simulink model "model1"  (R2023b)
settings: Solver=VariableStepAuto  StartTime=0.0  StopTime=8  RelTol=1e-3
model workspace (MAT data in the model file):
  T = Simulink.Parameter
  T.Value = 1
  T.DataType = 'auto'
  T.Complexity = 'real'
  T.Dimensions = [1 1]
  k = 1
  op = 2
settings Model: Creator=kacpe  LastModifiedBy=kacpe
settings DataIOCC: ReturnWorkspaceOutputs=off

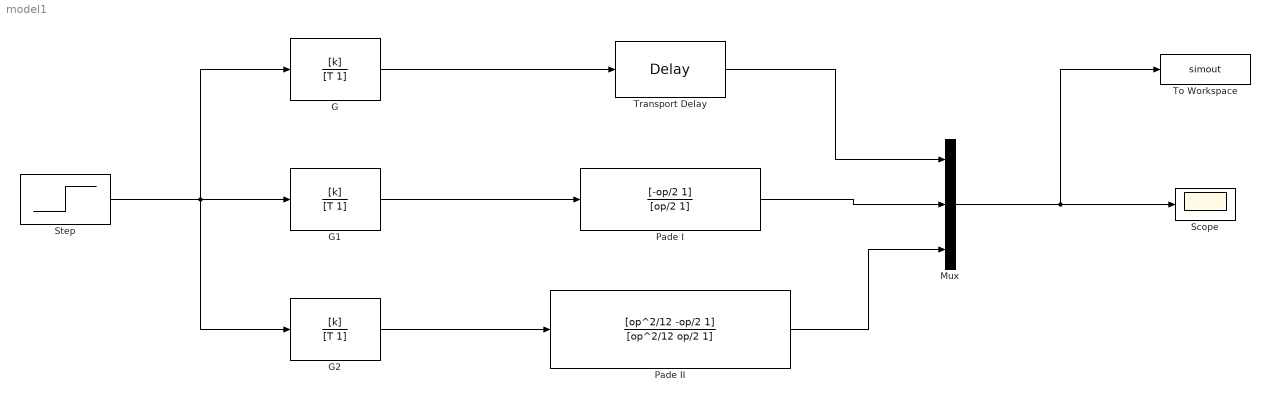
== system model1 ==
  G : TransferFcn  Numerator=[k]  Denominator=[T 1]
  G1 : TransferFcn  Numerator=[k]  Denominator=[T 1]
  G2 : TransferFcn  Numerator=[k]  Denominator=[T 1]
  Mux : Mux  Inputs=3
  Pade I : TransferFcn  Numerator=[-op/2 1]  Denominator=[op/2 1]
  Pade II : TransferFcn  Numerator=[op^2/12 -op/2 1]  Denominator=[op^2/12 op/2 1]
  Scope : Scope
  Step : Step  SampleTime=0
  To Workspace : ToWorkspace  VariableName=simout  SaveFormat=Timeseries  SampleTime=-1
  Transport Delay : TransportDelay
  wires:
  Step/1 -> G2/1, G1/1, G/1
  G/1 -> Transport Delay/1
  G1/1 -> Pade I/1
  G2/1 -> Pade II/1
  Mux/1 -> To Workspace/1, Scope/1
  Pade I/1 -> Mux/2
  Pade II/1 -> Mux/3
  Transport Delay/1 -> Mux/1
